simulink model "Qn8"  (R2022b)
settings: Solver=VariableStepAuto  StartTime=0.0  StopTime=10.0  RelTol=1e-3
settings Model: Creator=nmary  LastModifiedBy=nmary

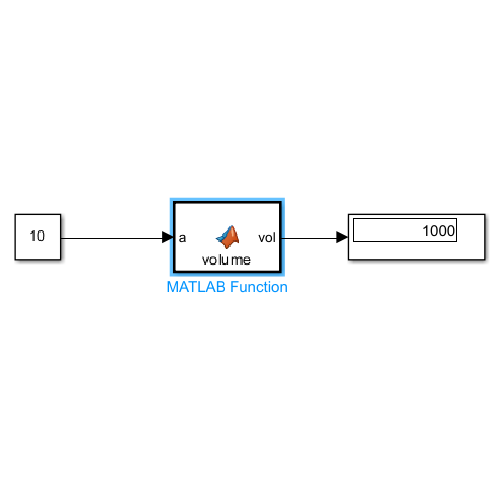
[thumbnail: Simulink's stored preview of the top-level diagram]
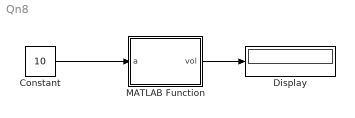
== system Qn8 ==
  Constant : Constant  Value=10
  Display : Display
  MATLAB Function : MATLAB Function  TreatAsAtomicUnit=on
  wires:
  Constant/1 -> MATLAB Function/1(a)
  MATLAB Function/1(vol) -> Display/1

== matlab function Qn8/MATLAB Function ==
  data: a input; vol output
% vloume of a cube

function vol = volume(a)

vol = a*a*a;
